simulink subsystem "Gcm"  (R2021b)
settings: Solver=VariableStepAuto  StartTime=0.0  StopTime=10.0  RelTol=1e-3
values from neighbouring files (symbols this model uses):
  Gcm_den_s0_SM_3 = 1/(Rm*Beq + nm*kt*km)    (= 1.00000097527)    [SM_Projet.m]
  Gcm_den_s1_SM_3 = 1/(Rm*Jeq)    (= 0.304488096074)    [SM_Projet.m]
  K_SM_3 = N*nm*kt    (= 0.33398001)    [SM_Projet.m]
settings Model: Creator=sama1402  LastModifiedBy=sama1402

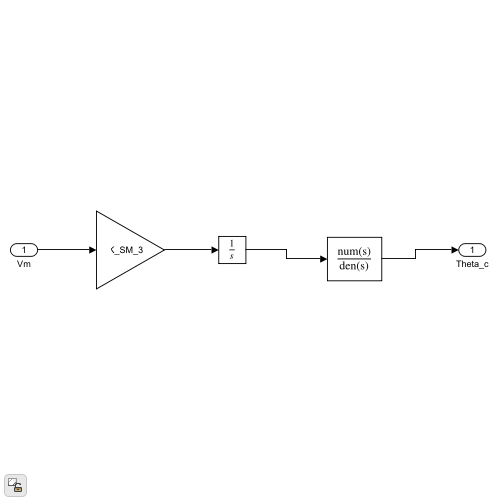
[thumbnail: Simulink's stored preview of the top-level diagram]
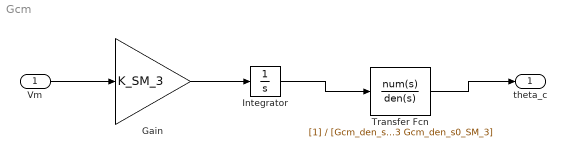
== system Gcm ==
  Vm : Inport
  Gain : Gain  Gain=K_SM_3
  Integrator : Integrator
  Transfer Fcn : TransferFcn  Denominator=[Gcm_den_s1_SM_3 Gcm_den_s0_SM_3]
  theta_c : Outport
  wires:
  Vm/1 -> Gain/1
  Gain/1 -> Integrator/1
  Integrator/1 -> Transfer Fcn/1
  Transfer Fcn/1 -> theta_c/1
